simulink model "gm_sla_VHT_HDL1080p_fil"  (R2015b)
settings: Solver=FixedStepDiscrete  SolverMode=SingleTasking  StartTime=0.0  StopTime=2200*1125*100  FixedStep=1  RelTol=1e-3
PreLoadFcn:
  | H = fspecial('unsharp')
undefined symbols (not defined in the file): gray
libraries: visionsinks x4, visionhdlio x2, fillib x1, visionconversions x1, visiongeotforms x1, dspvision x1
settings Model: SimulationMode=accelerator  Creator=yutengz  LastModifiedBy=amatsumo
settings DataIOCC: SaveFormat=Array
settings OptimizationCC: BlockReduction=off  BooleanDataType=off  ConditionallyExecuteInputs=off  DefaultParameterBehavior=Inlined
settings DebuggingCC: AlgebraicLoopMsg=error  SaveWithParameterizedLinksMsg=none  UnderspecifiedInitializationDetection=Classic  MergeDetectMultiDrivingBlocksExec=none  SignalResolutionControl=TryResolveAllWithWarning  InheritedTsInSrcMsg=none
settings HardwareCC: ProdBitPerPointer=32  ProdLargestAtomicFloat=None  ProdIntDivRoundTo=Undefined  ProdEndianess=Unspecified  ProdWordSize=32  ProdHWDeviceType=ASIC/FPGA->ASIC/FPGA  TargetUnknown=on  ProdEqTarget=off
settings GRTTargetCC: GeneratePreprocessorConditionals=Disable all
settings ConfigComp: CovModelRefEnable=Off  CovSFcnEnable=off

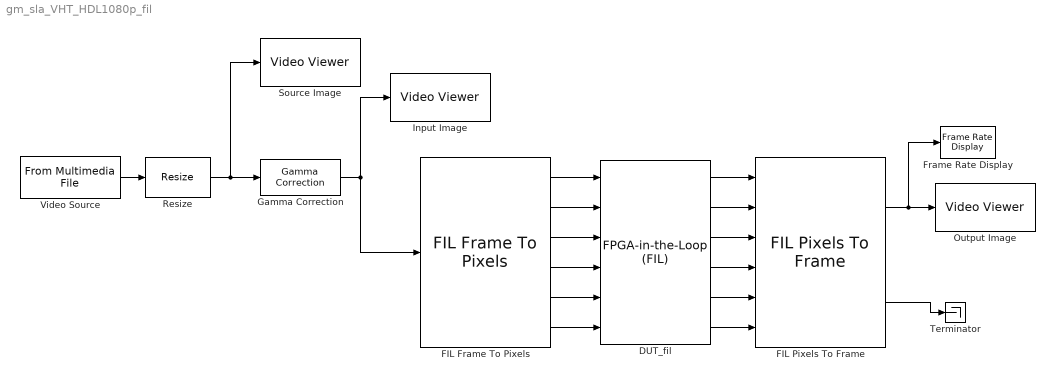
== system gm_sla_VHT_HDL1080p_fil ==
  DUT_fil : fillib/FPGA-in-the-Loop (FIL)  ForceInterfaceUpdate=0.90579
  FIL Frame To Pixels : visionhdlio/FIL Frame To Pixels  NumComponents=1  OutputVectorFormat=Frame  VideoFormat=1080p  ActivePixelsPerLine=32  ActiveVideoLines=18  TotalPixelsPerLine=42  TotalVideoLines=28  StartingActiveLine=6  FrontPorch=5  SampleTime=0
  FIL Pixels To Frame : visionhdlio/FIL Pixels To Frame  NumComponents=1  InputVectorFormat=Frame  VideoFormat=1080p  ActivePixelsPerLine=32  ActiveVideoLines=18  TotalPixelsPerLine=42  TotalVideoLines=28
  Frame Rate Display : visionsinks/Frame Rate Display  UpdateRate=10
  Gamma Correction : visionconversions/Gamma Correction  operation=De-gamma  gamma=2.2  linearSegment=on  breakPoint=0.018
  Input Image : visionsinks/Video Viewer  inputType=Obsolete7b  imagePorts=One multidimensional signal  useColorMap=off  colormapValue=gray(256)  specRange=off  minInputVal=0  maxInputVal=255  FigPos=[366 381 334 275]  AxisZoom=on  trueSizedOnce=off  OpenAtMdlStart=on  DefaultConfigurationName=vipscopes.VideoViewerScopeCfg
  Output Image : visionsinks/Video Viewer  inputType=Obsolete7b  imagePorts=One multidimensional signal  useColorMap=off  colormapValue=gray(256)  specRange=off  minInputVal=0  maxInputVal=255  FigPos=[709 384 334 275]  AxisZoom=on  trueSizedOnce=off  OpenAtMdlStart=on  DefaultConfigurationName=vipscopes.VideoViewerScopeCfg
  Resize : visiongeotforms/Resize  specify=Number of output rows and columns  rfactor=[200 150]  outCols=25  outRows=25  outRowsCols=[1080 1920]  interp_method=Bilinear  antialias=on  useROI=off  roiFlag=off  prodOutputMode=Binary point scaling  prodOutputWordLength=32  prodOutputFracLength=10  roundingMode=Nearest  overflowMode=on
  Source Image : visionsinks/Video Viewer  inputType=Obsolete7b  imagePorts=One multidimensional signal  useColorMap=off  colormapValue=gray(256)  specRange=off  minInputVal=0  maxInputVal=255  FigPos=[21 379 334 275]  AxisZoom=on  trueSizedOnce=off  OpenAtMdlStart=on  DefaultConfigurationName=vipscopes.VideoViewerScopeCfg
  Terminator : Terminator
  Video Source : dspvision/From Multimedia File  inputFilename=rhinos.avi  loop=on  numPlays=inf  outputStreams=Video only  videoDataType=uint8  audioDataType=int16  inheritSampleTime=off  userDefinedSampleTime="1125*2200  %402*324"  noAudioOutput=off  isIntensityVideo=off  fourcc=Intensity  colorVideoFormat=One multidimensional signal  outputEOF=off  dataOrg=Column-major  audioFrameSize=1024  computeAudioFrameSize=off  outSamplingMode=Sample based
  wires:
  Video Source/1 -> Resize/1
  FIL Pixels To Frame/1 -> Frame Rate Display/1, Output Image/1
  FIL Pixels To Frame/2 -> Terminator/1
  Gamma Correction/1 -> FIL Frame To Pixels/1, Input Image/1
  Resize/1 -> Source Image/1, Gamma Correction/1
  FIL Frame To Pixels/1 -> DUT_fil/1
  FIL Frame To Pixels/2 -> DUT_fil/2
  FIL Frame To Pixels/3 -> DUT_fil/3
  FIL Frame To Pixels/4 -> DUT_fil/4
  FIL Frame To Pixels/5 -> DUT_fil/5
  FIL Frame To Pixels/6 -> DUT_fil/6
  DUT_fil/1 -> FIL Pixels To Frame/1
  DUT_fil/2 -> FIL Pixels To Frame/2
  DUT_fil/3 -> FIL Pixels To Frame/3
  DUT_fil/4 -> FIL Pixels To Frame/4
  DUT_fil/5 -> FIL Pixels To Frame/5
  DUT_fil/6 -> FIL Pixels To Frame/6
